simulink model "Modell_PT1_mit_Winkel_linear_verteilteParam"  (R2016b)
settings: Solver=FixedStepAuto  StartTime=0.0  StopTime=10.0  FixedStep=1e-3  RelTol=1e-3
libraries: simulink x2
settings Model: Creator=nicol  LastModifiedBy=nicol
settings DataIOCC: ReturnWorkspaceOutputs=on
settings SFSimCC: SimUseLocalCustomCode=on
settings RTWCC: RTWUseLocalCustomCode=on

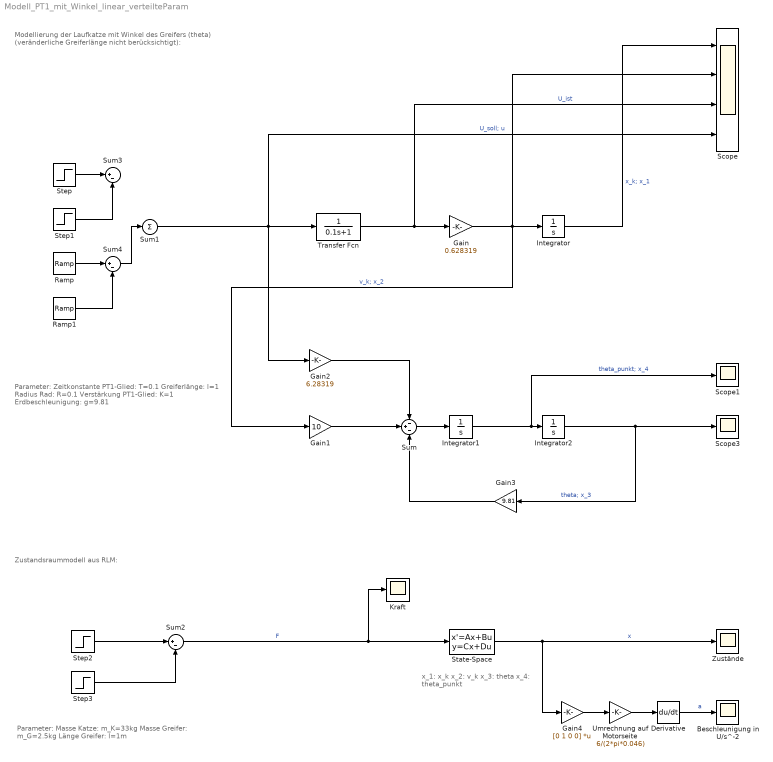
== system Modell_PT1_mit_Winkel_linear_verteilteParam ==
  note: x_1: x_k
      | x_2: v_k
      | x_3: theta
      | x_4: theta_punkt
  note: Zustandsraummodell aus RLM:
  note: Modellierung der Laufkatze mit Winkel des Greifers (theta) (veränderliche Greiferlänge nicht berücksichtigt):
  note: Parameter:
      | Zeitkonstante PT1-Glied: T=0.1
      | Greiferlänge: l=1
      | Radius Rad: R=0.1
      | Verstärkung PT1-Glied: K=1
      | Erdbeschleunigung: g=9.81
  note: Parameter:
      | Masse Katze: m_K=33kg
      | Masse Greifer: m_G=2.5kg
      | Länge Greifer: l=1m
  Beschleunigung in U/s^-2 : Scope
  Derivative : Derivative
  Gain : Gain  Gain=0.628319
  Gain1 : Gain  Gain=10
  Gain2 : Gain  Gain=6.28319
  Gain3 : Gain  Gain=9.81
  Gain4 : Gain  Gain=[0 1 0 0]  Multiplication=Matrix(K*u)
  Integrator : Integrator
  Integrator1 : Integrator
  Integrator2 : Integrator
  Kraft : Scope
  Ramp : simulink/Sources/Ramp  slope=0.1  start=1  X0=0
  Ramp1 : simulink/Sources/Ramp  slope=0.1  start=5  X0=0
  Scope : Scope  NumInputPorts=4
  Scope1 : Scope
  Scope3 : Scope
  State-Space : StateSpace  A=[0 1 0 0; 0 0 0.743182 0; 0 0 0 1; 0 0 -10.553182 0]  B=[0; 0.030303; 0; -0.030303]  C=[1 0 0 0; 0 1 0 0; 0 0 1 0; 0 0 0 1]  D=[0; 0; 0; 0]  X0=0
  Step : Step  SampleTime=0
  Step1 : Step  Time=4  SampleTime=0
  Step2 : Step  After=52.23  SampleTime=0
  Step3 : Step  Time=5  After=52.23  SampleTime=0
  Sum : Sum  Inputs=-+-
  Sum1 : Sum  Inputs=|+|
  Sum2 : Sum  Inputs=|+-
  Sum3 : Sum  Inputs=|+-
  Sum4 : Sum  Inputs=|+-
  Transfer Fcn : TransferFcn  Denominator=[0.1,1]
  "Umrechnung auf Motorseite " : Gain  Gain=6/(2*pi*0.046)
  Zustände : Scope
  wires:
  Transfer Fcn/1 -> Scope/3, Gain/1  "U_ist"
  Gain/1 -> Scope/2, Integrator/1, Gain1/1  "v_k; x_2"
  Integrator/1 -> Scope/1  "x_k; x_1"
  Gain2/1 -> Sum/1
  Sum/1 -> Integrator1/1
  Integrator1/1 -> Scope1/1, Integrator2/1  "theta_punkt; x_4"
  Integrator2/1 -> Gain3/1, Scope3/1  "theta; x_3"
  Gain3/1 -> Sum/3
  Gain1/1 -> Sum/2
  Sum1/1 -> Scope/4, Transfer Fcn/1, Gain2/1  "U_soll; u"
  State-Space/1 -> Gain4/1, Zustände/1  "x"
  Step3/1 -> Sum2/2
  Step2/1 -> Sum2/1
  Sum2/1 -> Kraft/1, State-Space/1  "F"
  Step/1 -> Sum3/1
  Step1/1 -> Sum3/2
  Ramp/1 -> Sum4/1
  Ramp1/1 -> Sum4/2
  Sum4/1 -> Sum1/1
  Derivative/1 -> Beschleunigung in U/s^-2/1  "a"
  "Umrechnung auf Motorseite "/1 -> Derivative/1
  Gain4/1 -> "Umrechnung auf Motorseite "/1
